simulink model "model_thumb_smc_mb"  (R2025b)
settings: Solver=ode4  StartTime=0.0  StopTime=15  FixedStep=0.0005  RelTol=1e-3
settings Model: Creator=ACER  LastModifiedBy=ACER

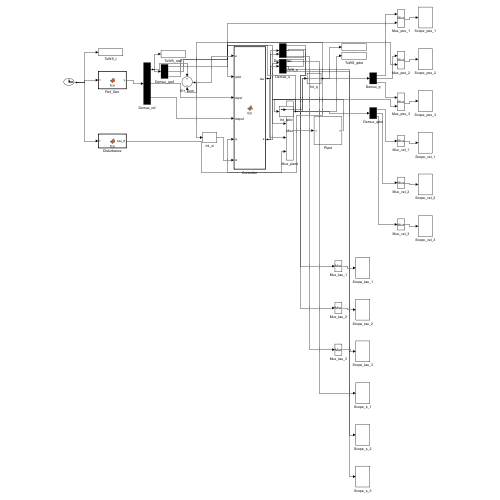
[thumbnail: Simulink's stored preview of the top-level diagram]
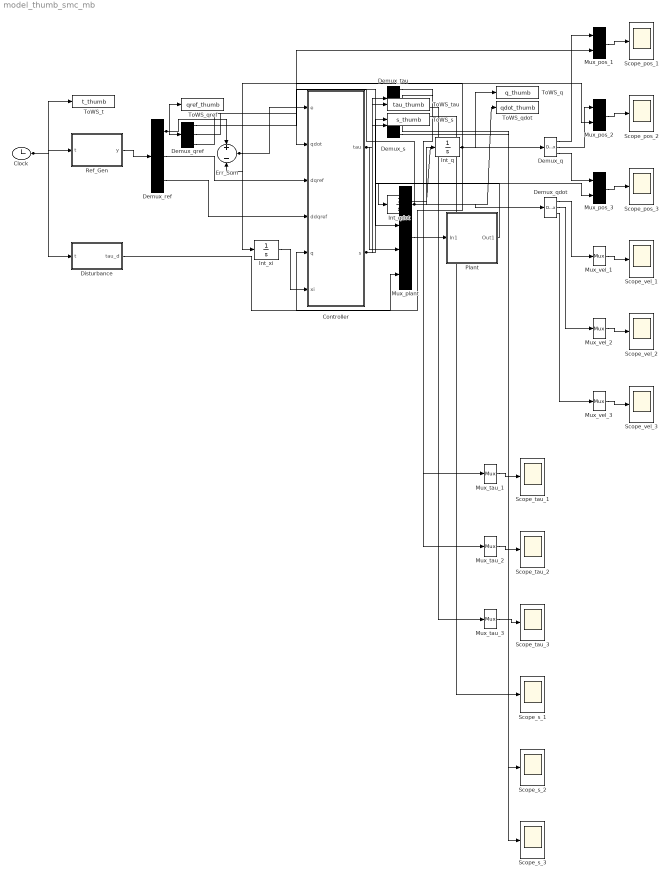
== system model_thumb_smc_mb ==
  Clock : Clock
  Controller : MATLAB Function  TreatAsAtomicUnit=on
  Demux_q : Demux  Outputs=3
  Demux_qdot : Demux  Outputs=3
  Demux_qref : Demux  Outputs=3
  Demux_ref : Demux  Outputs=[3 3 3]
  Demux_s : Demux  Outputs=3
  Demux_tau : Demux  Outputs=3
  Disturbance : MATLAB Function  TreatAsAtomicUnit=on
  Err_Sum : Sum  Inputs=+-
  Int_q : Integrator  InitialCondition=[0.45; 0.60; 0.30]
  Int_qdot : Integrator  InitialCondition=[0; 0; 0]
  Int_xi : Integrator  InitialCondition=[0; 0; 0]
  Mux_plant : Mux
  Mux_pos_1 : Mux  Inputs=2
  Mux_pos_2 : Mux  Inputs=2
  Mux_pos_3 : Mux  Inputs=2
  Mux_tau_1 : Mux  Inputs=1
  Mux_tau_2 : Mux  Inputs=1
  Mux_tau_3 : Mux  Inputs=1
  Mux_vel_1 : Mux  Inputs=1
  Mux_vel_2 : Mux  Inputs=1
  Mux_vel_3 : Mux  Inputs=1
  Plant : Subsystem
  Ref_Gen : MATLAB Function  TreatAsAtomicUnit=on
  Scope_pos_1 : Scope
  Scope_pos_2 : Scope
  Scope_pos_3 : Scope
  Scope_s_1 : Scope
  Scope_s_2 : Scope
  Scope_s_3 : Scope
  Scope_tau_1 : Scope
  Scope_tau_2 : Scope
  Scope_tau_3 : Scope
  Scope_vel_1 : Scope
  Scope_vel_2 : Scope
  Scope_vel_3 : Scope
  ToWS_q : ToWorkspace  VariableName=q_thumb
  ToWS_qdot : ToWorkspace  VariableName=qdot_thumb
  ToWS_qref : ToWorkspace  VariableName=qref_thumb
  ToWS_s : ToWorkspace  VariableName=s_thumb
  ToWS_t : ToWorkspace  VariableName=t_thumb
  ToWS_tau : ToWorkspace  VariableName=tau_thumb
  wires:
  Clock/1 -> Ref_Gen/1(t), Disturbance/1(t), ToWS_t/1
  Ref_Gen/1(y) -> Demux_ref/1
  Demux_ref/1 -> Err_Sum/1, ToWS_qref/1, Demux_qref/1
  Demux_ref/2 -> Controller/3(dqref)
  Demux_ref/3 -> Controller/4(ddqref)
  Err_Sum/1 -> Controller/1(e), Int_xi/1
  Int_xi/1 -> Controller/6(xi)
  Plant/1(Out1) -> Int_qdot/1
  Int_qdot/1 -> Int_q/1, Controller/2(qdot), Mux_plant/2, ToWS_qdot/1, Demux_qdot/1
  Int_q/1 -> Err_Sum/2, Controller/5(q), Mux_plant/1, ToWS_q/1, Demux_q/1
  Controller/1(tau) -> Mux_plant/3, ToWS_tau/1, Demux_tau/1
  Controller/2(s) -> ToWS_s/1, Demux_s/1
  Disturbance/1(tau_d) -> Mux_plant/4
  Mux_plant/1 -> Plant/1(In1)
  Demux_q/1 -> Mux_pos_1/1
  Demux_qref/1 -> Mux_pos_1/2
  Mux_pos_1/1 -> Scope_pos_1/1
  Demux_qdot/1 -> Mux_vel_1/1
  Mux_vel_1/1 -> Scope_vel_1/1
  Demux_tau/1 -> Mux_tau_1/1
  Mux_tau_1/1 -> Scope_tau_1/1
  Demux_s/1 -> Scope_s_1/1
  Demux_q/2 -> Mux_pos_2/1
  Demux_qref/2 -> Mux_pos_2/2
  Mux_pos_2/1 -> Scope_pos_2/1
  Demux_qdot/2 -> Mux_vel_2/1
  Mux_vel_2/1 -> Scope_vel_2/1
  Demux_tau/2 -> Mux_tau_2/1
  Mux_tau_2/1 -> Scope_tau_2/1
  Demux_s/2 -> Scope_s_2/1
  Demux_q/3 -> Mux_pos_3/1
  Demux_qref/3 -> Mux_pos_3/2
  Mux_pos_3/1 -> Scope_pos_3/1
  Demux_qdot/3 -> Mux_vel_3/1
  Mux_vel_3/1 -> Scope_vel_3/1
  Demux_tau/3 -> Mux_tau_3/1
  Mux_tau_3/1 -> Scope_tau_3/1
  Demux_s/3 -> Scope_s_3/1

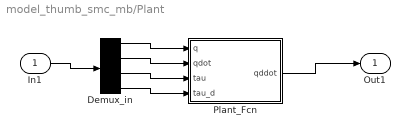
== system model_thumb_smc_mb/Plant ==
  In1 : Inport
  Demux_in : Demux  Outputs=[3 3 3 3]
  Plant_Fcn : MATLAB Function  TreatAsAtomicUnit=on
  Out1 : Outport
  wires:
  In1/1 -> Demux_in/1
  Demux_in/1 -> Plant_Fcn/1(q)
  Demux_in/2 -> Plant_Fcn/2(qdot)
  Demux_in/3 -> Plant_Fcn/3(tau)
  Demux_in/4 -> Plant_Fcn/4(tau_d)
  Plant_Fcn/1(qddot) -> Out1/1

== matlab function model_thumb_smc_mb/Controller ==
  data: e input; tau output; qdot input; dqref input; ddqref input; q input; xi input; s output
function [tau, s] = fcn(e, qdot, dqref, ddqref, q, xi)
Lambda = diag([8, 7, 8]);
K      = diag([0.012, 0.008, 0.005]);
delta  = 0.03;
eq_t  = -e;
deq_t = qdot - dqref;
s     = deq_t + Lambda*eq_t + 0*xi;
qdot_r  = dqref  - Lambda*eq_t;
qddot_r = ddqref - Lambda*deq_t;
r1=0.050; r2=0.035; r3=0.025;
m1=0.015; m2=0.010; m3=0.006;
J1=(1/3).*m1.*r1.^2; J2=(1/3).*m2.*r2.^2; J3=(1/3).*m3.*r3.^2;
c1=r1./2; c2=r2./2; c3=r3./2; g=9.81;
q1=q(1); q2=q(2); q3=q(3);
M11=J1+J2+J3+m1.*c1.^2+m2.*(r1.^2+c2.^2+2.*r1.*c2.*cos(q2))+m3.*(r1.^2+r2.^2+c3.^2+2.*r1.*r2.*cos(q2)+2.*r1.*c3.*cos(q2+q3)+2.*r2.*c3.*cos(q3));
M22=J2+J3+m2.*c2.^2+m3.*(r2.^2+c3.^2+2.*r2.*c3.*cos(q3));
M33=J3+m3.*c3.^2;
M12=J2+J3+m2.*(c2.^2+r1.*c2.*cos(q2))+m3.*(r2.^2+c3.^2+r1.*r2.*cos(q2)+r1.*c3.*cos(q2+q3)+2.*r2.*c3.*cos(q3));
M13=J3+m3.*(c3.^2+r1.*c3.*cos(q2+q3)+r2.*c3.*cos(q3));
M23=J3+m3.*(c3.^2+r2.*c3.*cos(q3));
M=[M11 M12 M13; M12 M22 M23; M13 M23 M33];
a2=m2.*r1.*c2.*sin(q2)+m3.*(r1.*r2.*sin(q2)+r1.*c3.*sin(q2+q3));
b3=m3.*r2.*c3.*sin(q3);
p3=m3.*r1.*c3.*sin(q2+q3);
qr1=qdot_r(1); qr2=qdot_r(2); qr3=qdot_r(3);
C1=-2.*a2.*qr1.*qr2 - a2.*qr2.^2 - 2.*(p3+b3).*(qr1+qr2).*qr3 - (p3+b3).*qr3.^2;
C2= a2.*qr1.^2 - 2.*b3.*(qr1+qr2).*qr3 - b3.*qr3.^2;
C3= p3.*qr1.^2 + b3.*(qr1+qr2).^2;
Cv_r=[C1; C2; C3];
s1=sin(q1); s12=sin(q1+q2); s123=sin(q1+q2+q3);
Gv=[g.*(m1.*c1.*s1+m2.*(r1.*s1+c2.*s12)+m3.*(r1.*s1+r2.*s12+c3.*s123));
    g.*(m2.*c2.*s12+m3.*(r2.*s12+c3.*s123));
    g.*m3.*c3.*s123];
tau_eq = M*qddot_r + Cv_r + Gv;
tau_sw = -K*sat_layer(s, delta);
tau    = tau_eq + tau_sw;
end

function y = sat_layer(s, delta)
y = zeros(3,1);
for i = 1:3
    if abs(s(i)) < delta, y(i) = s(i)./delta; else, y(i) = sign(s(i)); end
end
end

== matlab function model_thumb_smc_mb/Ref_Gen ==
  data: t input; y output
function y = fcn(t)
q0 = [0.45; 0.60; 0.30];
qf = [1.00; 0.80; 0.40];
dq = q0 - qf;
e1 = exp(-t);  e4 = exp(-4*t);
qref   = qf + (4/3).*dq.*e1 - (1/3).*dq.*e4;
dqref  =    - (4/3).*dq.*e1 + (4/3).*dq.*e4;
ddqref =      (4/3).*dq.*e1 - (16/3).*dq.*e4;
y = [qref; dqref; ddqref];
end

== matlab function model_thumb_smc_mb/Disturbance ==
  data: t input; tau_d output
function tau_d = fcn(t)
tau_d = [0.008.*sin(t)     + 0.002.*sin(200.*pi.*t);
         0.005.*cos(2.*t)   + 0.002.*sin(200.*pi.*t);
         0.003.*sin(0.5.*t) + 0.001.*sin(200.*pi.*t)];
end

== matlab function model_thumb_smc_mb/Plant/Plant_Fcn ==
  data: q input; qddot output; qdot input; tau input; tau_d input
function qddot = fcn(q, qdot, tau, tau_d)
q1=q(1); q2=q(2); q3=q(3);
qd1=qdot(1); qd2=qdot(2); qd3=qdot(3);
r1=0.050; r2=0.035; r3=0.025;
m1=0.015; m2=0.010; m3=0.006;
J1=(1/3).*m1.*r1.^2; J2=(1/3).*m2.*r2.^2; J3=(1/3).*m3.*r3.^2;
c1=r1./2; c2=r2./2; c3=r3./2; g=9.81;
M11=J1+J2+J3+m1.*c1.^2+m2.*(r1.^2+c2.^2+2.*r1.*c2.*cos(q2))+m3.*(r1.^2+r2.^2+c3.^2+2.*r1.*r2.*cos(q2)+2.*r1.*c3.*cos(q2+q3)+2.*r2.*c3.*cos(q3));
M22=J2+J3+m2.*c2.^2+m3.*(r2.^2+c3.^2+2.*r2.*c3.*cos(q3));
M33=J3+m3.*c3.^2;
M12=J2+J3+m2.*(c2.^2+r1.*c2.*cos(q2))+m3.*(r2.^2+c3.^2+r1.*r2.*cos(q2)+r1.*c3.*cos(q2+q3)+2.*r2.*c3.*cos(q3));
M13=J3+m3.*(c3.^2+r1.*c3.*cos(q2+q3)+r2.*c3.*cos(q3));
M23=J3+m3.*(c3.^2+r2.*c3.*cos(q3));
M=[M11 M12 M13; M12 M22 M23; M13 M23 M33];
a2=m2.*r1.*c2.*sin(q2)+m3.*(r1.*r2.*sin(q2)+r1.*c3.*sin(q2+q3));
b3=m3.*r2.*c3.*sin(q3);
p3=m3.*r1.*c3.*sin(q2+q3);
C1=-2.*a2.*qd1.*qd2 - a2.*qd2.^2 - 2.*(p3+b3).*(qd1+qd2).*qd3 - (p3+b3).*qd3.^2;
C2= a2.*qd1.^2 - 2.*b3.*(qd1+qd2).*qd3 - b3.*qd3.^2;
C3= p3.*qd1.^2 + b3.*(qd1+qd2).^2;
Cv=[C1; C2; C3];
s1=sin(q1); s12=sin(q1+q2); s123=sin(q1+q2+q3);
Gv=[g.*(m1.*c1.*s1+m2.*(r1.*s1+c2.*s12)+m3.*(r1.*s1+r2.*s12+c3.*s123));
    g.*(m2.*c2.*s12+m3.*(r2.*s12+c3.*s123));
    g.*m3.*c3.*s123];
qddot = M \ (tau + tau_d - Cv - Gv);
end
